simulink model "pulse_detector_ipcore"  (R2022b)
settings: Solver=FixedStepDiscrete  StartTime=0.0  StopTime=SimTime  RelTol=1e-3
InitFcn:
  | pulse_detector_init
undefined symbols (not defined in the file): CorrFilter, detectDelay, filterLatency, outputLength, preDetectDelay, RxSignal, threshold, WindowLen
libraries: dspsrcs4 x2, simulink x2, hdlsllib x2, dsphdlfiltering2 x1
settings Model: DataTypeOverride=Off  Creator=cchung  LastModifiedBy=bsingh
settings SolverCC: AlgebraicLoopSolver=TrustRegion
settings DataIOCC: SaveOutput=off  SaveTime=off
settings OptimizationCC: BlockReduction=off  ConditionallyExecuteInputs=off  DefaultParameterBehavior=Inlined  InheritOutputTypeSmallerThanSingle=on
settings DebuggingCC: AlgebraicLoopMsg=error  SingleTaskRateTransMsg=error  UnconnectedInputMsg=warning  UnconnectedOutputMsg=warning  UnconnectedLineMsg=warning  PregeneratedLibrarySubsystemCodeDiagnostic=none  SFMachineParentedDataDiag=warning  ArithmeticOperatorsInVariantConditions=warning
settings HardwareCC: ProdBitPerPointer=32  ProdBitPerSizeT=32  ProdBitPerPtrDiffT=32  ProdLargestAtomicFloat=None  ProdIntDivRoundTo=Undefined  ProdEndianess=Unspecified  ProdWordSize=32  ProdHWDeviceType=ASIC/FPGA->ASIC/FPGA  TargetBitPerPointer=64  TargetBitPerSizeT=64  TargetBitPerPtrDiffT=64  TargetLongLongMode=on  TargetIntDivRoundTo=Zero  TargetEndianess=LittleEndian  TargetWordSize=64  TargetHWDeviceType=Custom Processor->MATLAB Host Computer  ProdEqTarget=off
settings ModelReferenceCC: EnableRefExpFcnMdlSchedulingChecks=on
settings SFSimCC: SimUseLocalCustomCode=off  CustomCodeUndefinedFunction=UseInterfaceOnly
settings RTWCC: RTWUseLocalCustomCode=off  DLArmComputeVersion=19.05

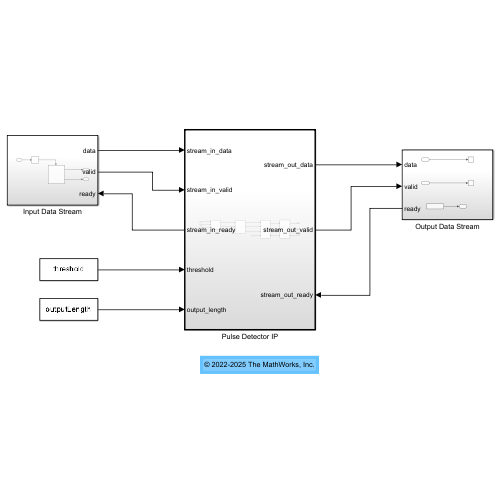
[thumbnail: Simulink's stored preview of the top-level diagram]
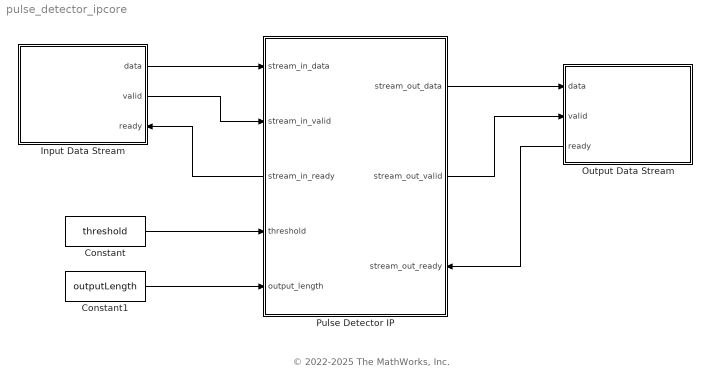
== system pulse_detector_ipcore ==
  note: © 2022-2025 The MathWorks, Inc.
  Constant : Constant  Value=threshold  OutDataTypeStr=Inherit: Inherit via back propagation  SampleTime=-1
  Constant1 : Constant  Value=outputLength  OutDataTypeStr=Inherit: Inherit via back propagation  SampleTime=-1
  Input Data Stream : Subsystem
      settings: PortSchema="{\"entries\":[{\"content\":{\"sides\":[{\"content\":{\"connectorIds\":[]},\"type\":\"ConnectorPlacement.EquallySpacedRectSide\",\"uuid\":\"cdc84fa2-4977-4d94-8c19-111ba0106cbc\"},{\"content\":{\"connectorIds\":[\"Out1\",\"Out2\",\"In1\"],\"side\":\"RIGHT\"},\"type\":\"ConnectorPlacement.EquallySpacedRectSide\",\"uuid\":\"2fd96718-903f-4027-b1fa-6a485b00905e\"},{\"content\":{\"connectorIds\":[],\"side\":\"TOP\"},\"type\":\"ConnectorPlacement.EquallySpacedRectSide\",\"uuid\":\"cf182822-3d09-48e1-9c4e-b73bc2793708\"}]},\"type\":\"ConnectorPlacement.EquallySpacedConnector\",\"uuid\":\"1b8b24a2-ceab-4874-8729-325ab0f09acf\"}],\"packageUris\":[\"http://schema.mathworks.com/mf0/Connector/R2020b\"],\"version\":\"1.0\"}"
  Output Data Stream : Subsystem
      settings: PortSchema="{\"entries\":[{\"content\":{\"sides\":[{\"content\":{\"connectorIds\":[\"In1\",\"In2\",\"Out1\"]},\"type\":\"ConnectorPlacement.EquallySpacedRectSide\",\"uuid\":\"11085236-e5c1-4710-acba-48068e52adda\"},{\"content\":{\"connectorIds\":[],\"side\":\"RIGHT\"},\"type\":\"ConnectorPlacement.EquallySpacedRectSide\",\"uuid\":\"8cfc156d-7e7f-429f-8966-4990f8d5cd25\"},{\"content\":{\"connectorIds\":[],\"side\":\"TOP\"},\"type\":\"ConnectorPlacement.EquallySpacedRectSide\",\"uuid\":\"ca29cfb1-febd-421b-b6f8-28f15e3b832e\"}]},\"type\":\"ConnectorPlacement.EquallySpacedConnector\",\"uuid\":\"5a1556ab-84d4-4563-9f2e-e478e0addac5\"}],\"packageUris\":[\"http://schema.mathworks.com/mf0/Connector/R2020b\"],\"version\":\"1.0\"}"
  Pulse Detector IP : Subsystem  TreatAsAtomicUnit=on
      settings: PortSchema="{\"entries\":[{\"content\":{\"sides\":[{\"content\":{\"connectorIds\":[\"In1\",\"In2\",\"Out3\",\"In3\",\"In4\"]},\"type\":\"ConnectorPlacement.EquallySpacedRectSide\",\"uuid\":\"710af840-d56b-4d7f-8589-87ad7b8a0450\"},{\"content\":{\"connectorIds\":[\"Out1\",\"Out2\",\"In5\"],\"side\":\"RIGHT\"},\"type\":\"ConnectorPlacement.EquallySpacedRectSide\",\"uuid\":\"c7ec467d-b6c0-4223-b16c-25f7adcce0e4\"},{\"content\":{\"connectorIds\":[],\"side\":\"TOP\"},\"type\":\"ConnectorPlacement.EquallySpacedRectSide\",\"uuid\":\"30e3ab0e-27a3-4a83-b548-bcb9b22a89cb\"}]},\"type\":\"ConnectorPlacement.EquallySpacedConnector\",\"uuid\":\"b361059a-4bfc-4799-959e-39b424b9a48b\"}],\"packageUris\":[\"http://schema.mathworks.com/mf0/Connector/R2020b\"],\"version\":\"1.0\"}"
  wires:
  Constant/1 -> Pulse Detector IP/3(threshold)
  Pulse Detector IP/3(stream_in_ready) -> Input Data Stream/1(ready)
  Constant1/1 -> Pulse Detector IP/4(output_length)
  Input Data Stream/1(data) -> Pulse Detector IP/1(stream_in_data)
  Input Data Stream/2(valid) -> Pulse Detector IP/2(stream_in_valid)
  Pulse Detector IP/1(stream_out_data) -> Output Data Stream/1(data)
  Pulse Detector IP/2(stream_out_valid) -> Output Data Stream/2(valid)
  Output Data Stream/1(ready) -> Pulse Detector IP/5(stream_out_ready)

== system pulse_detector_ipcore/Input Data Stream ==
  ready : Inport
  Subsystem : Subsystem
  Unit Delay : UnitDelay  SampleTime=-1  HasFrameUpgradeWarning=on
  data : Outport
  valid : Outport  Port=2
  wires:
  Subsystem/1(data) -> data/1
  Subsystem/2(valid) -> valid/1
  ready/1 -> Unit Delay/1
  Unit Delay/1 -> Subsystem/Enable

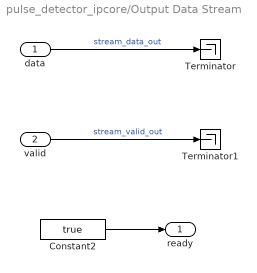
== system pulse_detector_ipcore/Output Data Stream ==
  data : Inport
  valid : Inport  Port=2
  Constant2 : Constant  Value=true  SampleTime=-1
  Terminator : Terminator
  Terminator1 : Terminator
  ready : Outport
  wires:
  Constant2/1 -> ready/1
  data/1 -> Terminator/1  "stream_data_out"
  valid/1 -> Terminator1/1  "stream_valid_out"

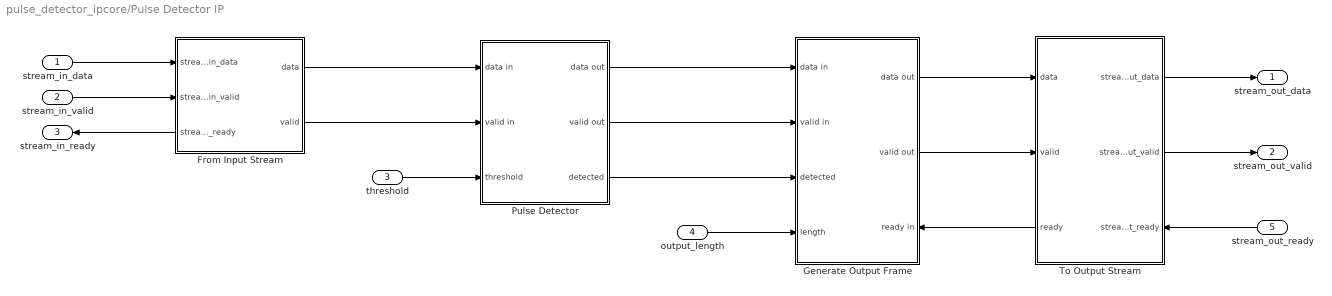
== system pulse_detector_ipcore/Pulse Detector IP ==
  stream_in_data : Inport
  stream_in_valid : Inport  Port=2
  threshold : Inport  Port=3
  output_length : Inport  Port=4
  stream_out_ready : Inport  Port=5
  From Input Stream : Subsystem
      settings: PortSchema="{\"entries\":[{\"content\":{\"sides\":[{\"content\":{\"connectorIds\":[\"In1\",\"In2\",\"Out3\"]},\"type\":\"ConnectorPlacement.EquallySpacedRectSide\",\"uuid\":\"5a70d6dd-43fd-4476-8df8-ae9cfc372135\"},{\"content\":{\"connectorIds\":[\"Out1\",\"Out2\"],\"side\":\"RIGHT\"},\"type\":\"ConnectorPlacement.EquallySpacedRectSide\",\"uuid\":\"8028c36d-bf46-4ae4-b540-6f6bfa5c14b3\"},{\"content\":{\"connectorIds\":[],\"side\":\"TOP\"},\"type\":\"ConnectorPlacement.EquallySpacedRectSide\",\"uuid\":\"1d4a1e8f-5e01-4fd1-be5f-3ade628adeeb\"}]},\"type\":\"ConnectorPlacement.EquallySpacedConnector\",\"uuid\":\"385ae01d-069b-45d2-add1-90b79875272d\"}],\"packageUris\":[\"http://schema.mathworks.com/mf0/Connector/R2020b\"],\"version\":\"1.0\"}"
  Generate Output Frame : Subsystem
      settings: PortSchema="{\"entries\":[{\"content\":{\"sides\":[{\"content\":{\"connectorIds\":[\"In1\",\"In2\",\"In3\",\"In4\"]},\"type\":\"ConnectorPlacement.EquallySpacedRectSide\",\"uuid\":\"6f09e145-48ee-41d2-bec3-6a733c9106b2\"},{\"content\":{\"connectorIds\":[\"Out1\",\"Out2\",\"In5\"],\"side\":\"RIGHT\"},\"type\":\"ConnectorPlacement.EquallySpacedRectSide\",\"uuid\":\"546a5f38-a809-4883-a76f-61cab94f6d84\"},{\"content\":{\"connectorIds\":[],\"side\":\"TOP\"},\"type\":\"ConnectorPlacement.EquallySpacedRectSide\",\"uuid\":\"11739b25-d16f-46c4-9eb7-ceb525177655\"}]},\"type\":\"ConnectorPlacement.EquallySpacedConnector\",\"uuid\":\"2379cc98-1392-4372-a564-c1eaf6dbd020\"}],\"packageUris\":[\"http://schema.mathworks.com/mf0/Connector/R2020b\"],\"version\":\"1.0\"}"
  Pulse Detector : Subsystem
  To Output Stream : Subsystem
      settings: PortSchema="{\"entries\":[{\"content\":{\"sides\":[{\"content\":{\"connectorIds\":[\"In1\",\"In2\",\"Out3\"]},\"type\":\"ConnectorPlacement.EquallySpacedRectSide\",\"uuid\":\"97942b52-de25-4521-8d66-ec2017a34e79\"},{\"content\":{\"connectorIds\":[\"Out1\",\"Out2\",\"In3\"],\"side\":\"RIGHT\"},\"type\":\"ConnectorPlacement.EquallySpacedRectSide\",\"uuid\":\"0e941ddc-855e-4920-a002-1054ec6cc8c6\"},{\"content\":{\"connectorIds\":[],\"side\":\"TOP\"},\"type\":\"ConnectorPlacement.EquallySpacedRectSide\",\"uuid\":\"8f802294-fdeb-49d3-9738-4cda18deb86a\"}]},\"type\":\"ConnectorPlacement.EquallySpacedConnector\",\"uuid\":\"22fe41de-4682-4463-b3e0-2e88c666c424\"}],\"packageUris\":[\"http://schema.mathworks.com/mf0/Connector/R2020b\"],\"version\":\"1.0\"}"
  stream_out_data : Outport
  stream_out_valid : Outport  Port=2
  stream_in_ready : Outport  Port=3
  wires:
  threshold/1 -> Pulse Detector/3(threshold)
  Pulse Detector/2(valid out) -> Generate Output Frame/2(valid in)
  Pulse Detector/3(detected) -> Generate Output Frame/3(detected)
  output_length/1 -> Generate Output Frame/4(length)
  Generate Output Frame/2(valid out) -> To Output Stream/2(valid)
  To Output Stream/3(ready) -> Generate Output Frame/5(ready in)
  Pulse Detector/1(data out) -> Generate Output Frame/1(data in)
  Generate Output Frame/1(data out) -> To Output Stream/1(data)
  stream_out_ready/1 -> To Output Stream/3(stream_out_ready)
  stream_in_data/1 -> From Input Stream/1(stream_in_data)
  stream_in_valid/1 -> From Input Stream/2(stream_in_valid)
  From Input Stream/1(data) -> Pulse Detector/1(data in)
  From Input Stream/2(valid) -> Pulse Detector/2(valid in)
  From Input Stream/3(stream_in_ready) -> stream_in_ready/1
  To Output Stream/1(stream_out_data) -> stream_out_data/1
  To Output Stream/2(stream_out_valid) -> stream_out_valid/1

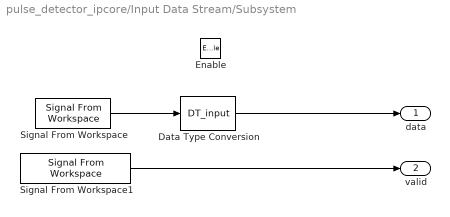
== system pulse_detector_ipcore/Input Data Stream/Subsystem ==
  Enable : EnablePort
  Data Type Conversion : DataTypeConversion  OutDataTypeStr=DT_input  RndMeth=Nearest
  Signal From Workspace : dspsrcs4/Signal From Workspace  X=RxSignal  Ts=1  nsamps=1  OutputAfterFinalValue=Setting to zero  ignoreOrWarnInputAndFrameLengths=off  OutputFrames=off
  Signal From Workspace1 : dspsrcs4/Signal From Workspace  X=true(size(RxSignal))  Ts=1  nsamps=1  OutputAfterFinalValue=Setting to zero  ignoreOrWarnInputAndFrameLengths=off  OutputFrames=off
  data : Outport
  valid : Outport  Port=2
  wires:
  Signal From Workspace/1 -> Data Type Conversion/1
  Data Type Conversion/1 -> data/1
  Signal From Workspace1/1 -> valid/1

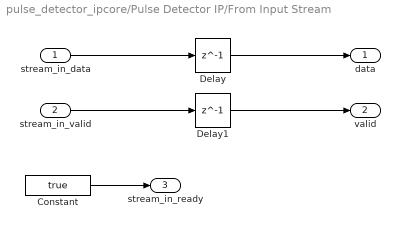
== system pulse_detector_ipcore/Pulse Detector IP/From Input Stream ==
  stream_in_data : Inport
  stream_in_valid : Inport  Port=2
  Constant : Constant  Value=true  SampleTime=-1
  Delay : Delay  DelayLength=1
  Delay1 : Delay  DelayLength=1
  data : Outport
  valid : Outport  Port=2
  stream_in_ready : Outport  Port=3
  wires:
  stream_in_valid/1 -> Delay1/1
  stream_in_data/1 -> Delay/1
  Constant/1 -> stream_in_ready/1
  Delay/1 -> data/1
  Delay1/1 -> valid/1

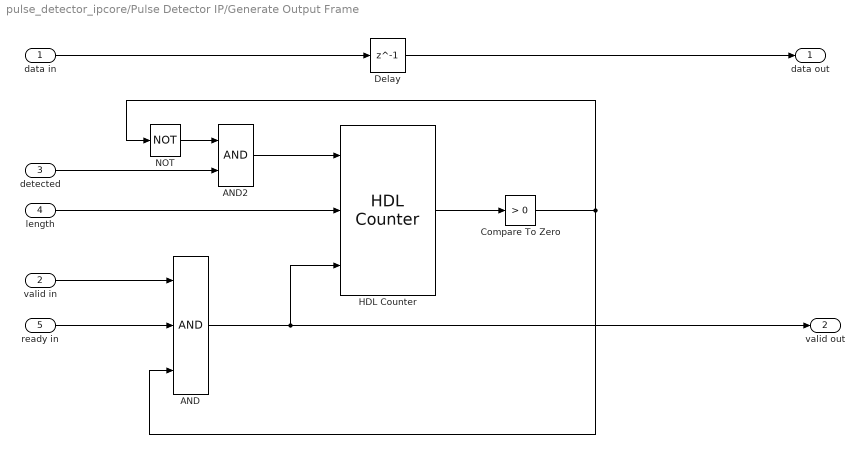
== system pulse_detector_ipcore/Pulse Detector IP/Generate Output Frame ==
  data in : Inport
  valid in : Inport  Port=2
  detected : Inport  Port=3
  length : Inport  Port=4
  ready in : Inport  Port=5
  AND : Logic  Inputs=3  IconShape=distinctive  AllPortsSameDT=off  OutDataTypeStr=boolean
  AND2 : Logic  IconShape=distinctive  AllPortsSameDT=off  OutDataTypeStr=boolean
  Compare To Zero : simulink/Logic and Bit Operations/Compare To Zero  relop=>  OutDataTypeStr=boolean
  Delay : Delay  DelayLength=1
  HDL Counter : hdlsllib/Sources/HDL Counter  CountType=Free running  CountInit=0  CountStep=-1  CountMax=25  CountFromType=Initial value  CountFrom=0  CountResetPort=off  CountLoadPort=on  CountEnbPort=on  CountDirPort=off  CountHitOutputPort=off  CountDataType=Unsigned  CountWordLen=32  CountFracLen=0  CountSampTime=1
  NOT : Logic  Operator=NOT  IconShape=distinctive  AllPortsSameDT=off  OutDataTypeStr=boolean
  data out : Outport
  valid out : Outport  Port=2
  wires:
  HDL Counter/1 -> Compare To Zero/1
  Compare To Zero/1 -> NOT/1, AND/3
  AND/1 -> HDL Counter/3, valid out/1
  valid in/1 -> AND/1
  ready in/1 -> AND/2
  length/1 -> HDL Counter/2
  AND2/1 -> HDL Counter/1
  NOT/1 -> AND2/1
  detected/1 -> AND2/2
  data in/1 -> Delay/1
  Delay/1 -> data out/1

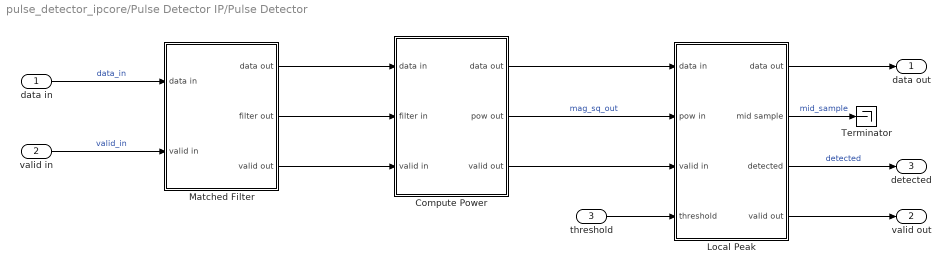
== system pulse_detector_ipcore/Pulse Detector IP/Pulse Detector ==
  data in : Inport
  valid in : Inport  Port=2
  threshold : Inport  Port=3
  Compute Power : Subsystem
  Local Peak : Subsystem
  Matched Filter : Subsystem
  Terminator : Terminator
  data out : Outport
  valid out : Outport  Port=2
  detected : Outport  Port=3
  wires:
  Local Peak/3(detected) -> detected/1  "detected"
  Compute Power/2(pow out) -> Local Peak/2(pow in)  "mag_sq_out"
  Local Peak/1(data out) -> data out/1
  Local Peak/4(valid out) -> valid out/1
  Compute Power/3(valid out) -> Local Peak/3(valid in)
  threshold/1 -> Local Peak/4(threshold)
  Compute Power/1(data out) -> Local Peak/1(data in)
  Local Peak/2(mid sample) -> Terminator/1  "mid_sample"
  data in/1 -> Matched Filter/1(data in)  "data_in"
  valid in/1 -> Matched Filter/2(valid in)  "valid_in"
  Matched Filter/2(filter out) -> Compute Power/2(filter in)
  Matched Filter/3(valid out) -> Compute Power/3(valid in)
  Matched Filter/1(data out) -> Compute Power/1(data in)

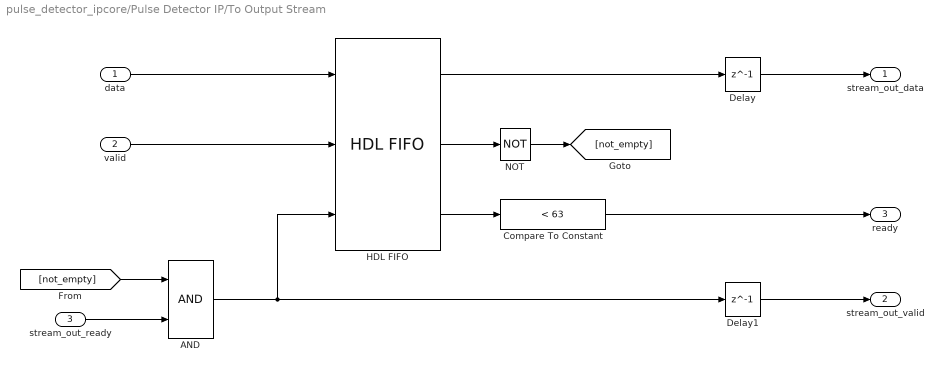
== system pulse_detector_ipcore/Pulse Detector IP/To Output Stream ==
  data : Inport
  valid : Inport  Port=2
  stream_out_ready : Inport  Port=3
  AND : Logic  IconShape=distinctive  AllPortsSameDT=off  OutDataTypeStr=boolean
  Compare To Constant : simulink/Logic and Bit Operations/Compare To Constant  relop=<  const=63  OutDataTypeStr=boolean
  Delay : Delay  DelayLength=1
  Delay1 : Delay  DelayLength=1
  HDL FIFO : hdlsllib/HDL RAMs/HDL FIFO  fifo_size=64  mode=FWFT  ratio=1  push_msg=Warning  pop_msg=Warning  show_empty=on  show_full=off  show_num=on  LabelModeActiveChoice_Mode=FWFT  rst_port=off
  NOT : Logic  Operator=NOT  IconShape=distinctive  AllPortsSameDT=off  OutDataTypeStr=boolean
  stream_out_data : Outport
  stream_out_valid : Outport  Port=2
  ready : Outport  Port=3
  wires:
  Delay/1 -> stream_out_data/1
  Compare To Constant/1 -> ready/1
  Delay1/1 -> stream_out_valid/1
  AND/1 -> Delay1/1, HDL FIFO/3
  valid/1 -> HDL FIFO/2
  HDL FIFO/2 -> NOT/1
  data/1 -> HDL FIFO/1
  stream_out_ready/1 -> AND/2
  HDL FIFO/1 -> Delay/1
  NOT/1 -> [not_empty]
  [not_empty] -> AND/1
  HDL FIFO/3 -> Compare To Constant/1

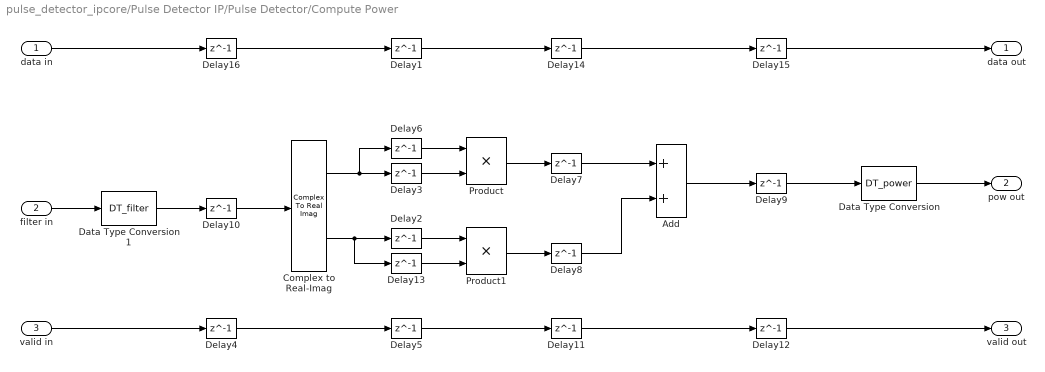
== system pulse_detector_ipcore/Pulse Detector IP/Pulse Detector/Compute Power ==
  data in : Inport
  filter in : Inport  Port=2
  valid in : Inport  Port=3
  Add : Sum
  Complex to Real-Imag : ComplexToRealImag
  Data Type Conversion : DataTypeConversion  OutDataTypeStr=DT_power  SaturateOnIntegerOverflow=off  RndMeth=Floor
  Data Type Conversion1 : DataTypeConversion  OutDataTypeStr=DT_filter  SaturateOnIntegerOverflow=off  RndMeth=Floor
  Delay{1..16} (16 alike) : Delay  DelayLength=1
  Product : Product
  Product1 : Product
  data out : Outport  VectorParamsAs1DForOutWhenUnconnected=off
  pow out : Outport  Port=2  VectorParamsAs1DForOutWhenUnconnected=off
  valid out : Outport  Port=3  VectorParamsAs1DForOutWhenUnconnected=off
  wires:
  Product/1 -> Delay7/1
  Add/1 -> Delay9/1
  filter in/1 -> Data Type Conversion1/1
  Data Type Conversion1/1 -> Delay10/1
  Data Type Conversion/1 -> pow out/1
  valid in/1 -> Delay4/1
  Delay4/1 -> Delay5/1
  Delay10/1 -> Complex to Real-Imag/1
  Delay3/1 -> Product/2
  Complex to Real-Imag/2 -> Delay2/1, Delay13/1
  Product1/1 -> Delay8/1
  Complex to Real-Imag/1 -> Delay6/1, Delay3/1
  Delay7/1 -> Add/1
  Delay8/1 -> Add/2
  Delay9/1 -> Data Type Conversion/1
  Delay5/1 -> Delay11/1
  Delay11/1 -> Delay12/1
  Delay12/1 -> valid out/1
  Delay1/1 -> Delay14/1
  Delay14/1 -> Delay15/1
  Delay15/1 -> data out/1
  data in/1 -> Delay16/1
  Delay6/1 -> Product/1
  Delay2/1 -> Product1/1
  Delay13/1 -> Product1/2
  Delay16/1 -> Delay1/1

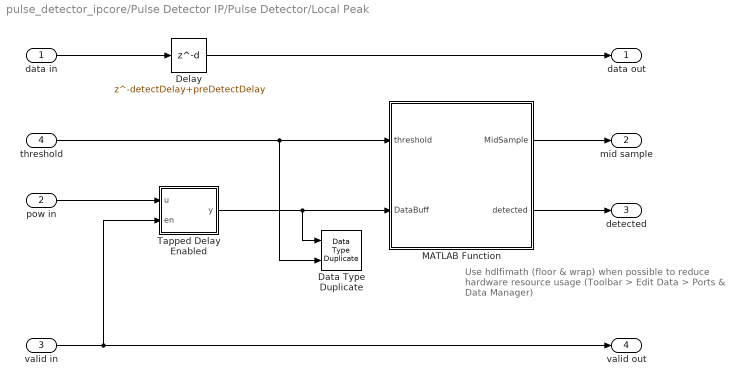
== system pulse_detector_ipcore/Pulse Detector IP/Pulse Detector/Local Peak ==
  note: Use hdlfimath (floor & wrap) when possible
      | to reduce hardware resource usage
      | (Toolbar > Edit Data > Ports & Data Manager)
  data in : Inport
  pow in : Inport  Port=2
  valid in : Inport  Port=3
  threshold : Inport  Port=4
  Data Type Duplicate : DataTypeDuplicate
  Delay : Delay  DelayLength=detectDelay+preDetectDelay
  MATLAB Function : MATLAB Function  TreatAsAtomicUnit=on
  Tapped Delay Enabled : Subsystem  mask(Tapped Delay Line Enabled){N=WindowLen, order=Oldest, outdim=1-D array}
      mask prompts: N "Number of delays:"; order "Order output vector starting with:"; outdim "Output dimensionality:"
      mask help: Delay a signal N sample periods and output all delay versions.
      mask TypeOptions order: Oldest | Newest
      mask TypeOptions outdim: 1-D array | Column vector (2-D) | Row vector (2-D)
      mask Display: fprintf('%d\nDelays',N);
  data out : Outport  VectorParamsAs1DForOutWhenUnconnected=off
  mid sample : Outport  Port=2  VectorParamsAs1DForOutWhenUnconnected=off
  detected : Outport  Port=3  VectorParamsAs1DForOutWhenUnconnected=off
  valid out : Outport  Port=4
  wires:
  pow in/1 -> Tapped Delay Enabled/1(u)
  Tapped Delay Enabled/1(y) -> Data Type Duplicate/1, MATLAB Function/2(DataBuff)
  threshold/1 -> Data Type Duplicate/2, MATLAB Function/1(threshold)
  MATLAB Function/1(MidSample) -> mid sample/1
  MATLAB Function/2(detected) -> detected/1
  valid in/1 -> valid out/1, Tapped Delay Enabled/2(en)
  data in/1 -> Delay/1
  Delay/1 -> data out/1

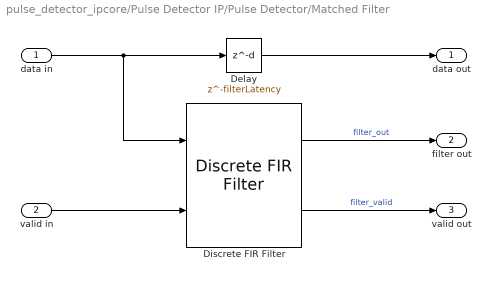
== system pulse_detector_ipcore/Pulse Detector IP/Pulse Detector/Matched Filter ==
  data in : Inport
  valid in : Inport  Port=2
  Delay : Delay  DelayLength=filterLatency
  Discrete FIR Filter : dsphdlfiltering2/Discrete FIR Filter  NumeratorSource=Property  Numerator=CorrFilter  NumeratorPrototype=[]  FilterStructure=Direct form systolic  SerializationOption=Minimum number of cycles between valid input samples  NumCycles=2  NumberOfMultipliers=2  SimulateUsing=Code generation  roundingMode=Floor  overflowMode=off  CoefficientsDataTypeStr=DT_coeff  ResetInputPort=off  HDLGlobalReset=off
  data out : Outport
  filter out : Outport  Port=2
  valid out : Outport  Port=3
  wires:
  Discrete FIR Filter/2 -> valid out/1  "filter_valid"
  data in/1 -> Discrete FIR Filter/1, Delay/1
  valid in/1 -> Discrete FIR Filter/2
  Discrete FIR Filter/1 -> filter out/1  "filter_out"
  Delay/1 -> data out/1

== system pulse_detector_ipcore/Pulse Detector IP/Pulse Detector/Local Peak/Tapped Delay Enabled ==
  u : Inport
  en : Inport  Port=2
  Reshape : Subsystem  Variant=on
  tapped_delay_impl : Subsystem
  y : Outport
  wires:
  Reshape/1(Out1) -> y/1
  tapped_delay_impl/1(y) -> Reshape/1(In1)
  u/1 -> tapped_delay_impl/1(u)
  en/1 -> tapped_delay_impl/2(en)

== system pulse_detector_ipcore/Pulse Detector IP/Pulse Detector/Local Peak/Tapped Delay Enabled/Reshape ==
  In1 : Inport
  "1D " : Subsystem  VariantControl=outdim == 1
  Column : Subsystem  VariantControl=outdim == 2
  Row : Subsystem  VariantControl=outdim == 3
  Out1 : Outport

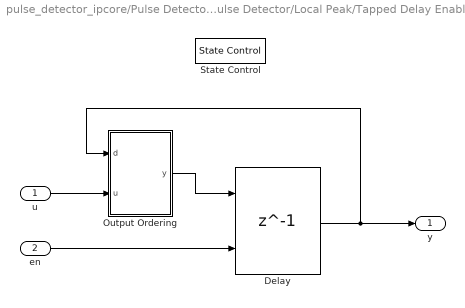
== system pulse_detector_ipcore/Pulse Detector IP/Pulse Detector/Local Peak/Tapped Delay Enabled/tapped_delay_impl ==
  u : Inport
  en : Inport  Port=2
  Delay : Delay  DelayLength=1  InitialCondition=zeros(N,1)  ShowEnablePort=on
      settings: InputPortMap=u0,e6
  Output Ordering : Subsystem  Variant=on
  State Control : StateControl  StateControl=Synchronous
  y : Outport
  wires:
  u/1 -> Output Ordering/2(u)
  Output Ordering/1(y) -> Delay/1
  Delay/1 -> y/1, Output Ordering/1(d)
  en/1 -> Delay/2

== system pulse_detector_ipcore/Pulse Detector IP/Pulse Detector/Local Peak/Tapped Delay Enabled/Reshape/1D  ==
  In1 : Inport
  Reshape : Reshape
  Out1 : Outport
  wires:
  In1/1 -> Reshape/1
  Reshape/1 -> Out1/1

== system pulse_detector_ipcore/Pulse Detector IP/Pulse Detector/Local Peak/Tapped Delay Enabled/Reshape/Column ==
  In1 : Inport
  Reshape : Reshape  OutputDimensionality=Column vector (2-D)
  Out1 : Outport
  wires:
  Reshape/1 -> Out1/1
  In1/1 -> Reshape/1

== system pulse_detector_ipcore/Pulse Detector IP/Pulse Detector/Local Peak/Tapped Delay Enabled/Reshape/Row ==
  In1 : Inport
  Reshape : Reshape  OutputDimensionality=Row vector (2-D)
  Out1 : Outport
  wires:
  In1/1 -> Reshape/1
  Reshape/1 -> Out1/1

== system pulse_detector_ipcore/Pulse Detector IP/Pulse Detector/Local Peak/Tapped Delay Enabled/tapped_delay_impl/Output Ordering ==
  d : Inport
  u : Inport  Port=2
  Newest : Subsystem  VariantControl=order == 2
  Oldest : Subsystem  VariantControl=order == 1
  y : Outport

== system pulse_detector_ipcore/Pulse Detector IP/Pulse Detector/Local Peak/Tapped Delay Enabled/tapped_delay_impl/Output Ordering/Newest ==
  u : Inport
  d : Inport  Port=2
  Selector : Selector  NumberOfDimensions=2  InputPortWidth=3  IndexOptions=Index vector (dialog),Index vector (dialog)  Indices=[1:N-1],1  OutputSizes=1,1
  Vector Concatenate : Concatenate
  y : Outport
  wires:
  Selector/1 -> Vector Concatenate/2
  u/1 -> Vector Concatenate/1
  Vector Concatenate/1 -> y/1
  d/1 -> Selector/1

== system pulse_detector_ipcore/Pulse Detector IP/Pulse Detector/Local Peak/Tapped Delay Enabled/tapped_delay_impl/Output Ordering/Oldest ==
  u : Inport
  d : Inport  Port=2
  Selector : Selector  NumberOfDimensions=2  InputPortWidth=3  IndexOptions=Index vector (dialog),Index vector (dialog)  Indices=[2:N],1  OutputSizes=1,1
  Vector Concatenate : Concatenate
  y : Outport
  wires:
  u/1 -> Vector Concatenate/2
  d/1 -> Selector/1
  Selector/1 -> Vector Concatenate/1
  Vector Concatenate/1 -> y/1

== matlab function pulse_detector_ipcore/Pulse Detector IP/Pulse Detector/Local Peak/MATLAB Function ==
  data: WindowLen parameter; threshold input; DataBuff input; MidSample output; detected output
% Hardware friendly implementation of peak finder
%
% Function inputs:
% * WindowLen - non-tunable parameter defined under Simulink->Edit Data
% * threhold  - input port (connected to constant)
% * DataBuff  - input port (buffering done using Simulink block)
%
% Function outputs:
% * "detected" is set when MidSample is local max

function [MidSample,detected] = fcn(WindowLen, threshold, DataBuff)
%#codegen


MidIdx = ceil(WindowLen/2);

% Compare each value in the window to the middle sample via subtraction
MidSample = DataBuff(MidIdx);
CompareOut = DataBuff - MidSample; % this is a vector

% if all values in the result are negative and the middle sample is
% greater than a threshold, it is a local max
if all(CompareOut <= 0) && (MidSample > threshold)
    detected = true;
else
    detected = false;
end
